simulink model "targetDice"  (R2020a)
settings: Solver=VariableStepAuto  StartTime=0.0  StopTime=20  RelTol=1e-3
model workspace (MAT data in the model file):
  d = [1  1  1  5  5  8; 2  2  3  3  6  6; 1  4  4  4  5  7; 2  2  6  6  7  8; 3  4  5  7  8  8]
  seed = 1234
libraries: simulink x1, rllib x1
settings Model: OrderedModelArguments=off  Creator=mtearle  LastModifiedBy=mtearle

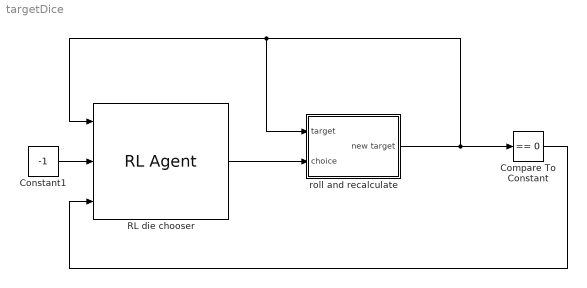
== system targetDice ==
  Compare To Constant : simulink/Logic and Bit Operations/Compare To Constant  relop===  const=0  OutDataTypeStr=boolean
  Constant1 : Constant  Value=-1
  RL die chooser : rllib/RL Agent  Agent=agent  ProvideReward=on  ProvideIsDone=on  ProvideCumRwd=off  TreatAsDirectFeedthrough=on  CollectLoggedSignals=on  CollectModelStates=on
  roll and recalculate : Subsystem
  wires:
  roll and recalculate/1(" new target") -> Compare To Constant/1, roll and recalculate/1(target), RL die chooser/1
  RL die chooser/1 -> roll and recalculate/2(choice)
  Constant1/1 -> RL die chooser/2
  Compare To Constant/1 -> RL die chooser/3

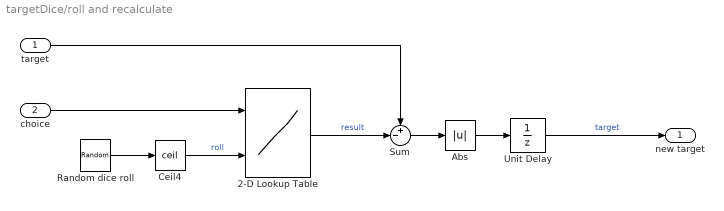
== system targetDice/roll and recalculate ==
  target : Inport
  choice : Inport  Port=2
  2-D Lookup Table : Lookup_n-D  BreakpointsSpecification=Even spacing  BreakpointsForDimension1=[1:3]  BreakpointsForDimension2=[1:3]  Table=d  InternalRulePriority=Speed  RndMeth=Simplest  InputSameDT=on
  Abs : Abs
  Ceil4 : Rounding  Operator=ceil
  Random dice roll : UniformRandomNumber  Minimum=0  Maximum=size(d,2)  Seed=seed  SampleTime=1
  Sum : Sum  Inputs=+-|
  Unit Delay : UnitDelay  InitialCondition=randi(20)  HasFrameUpgradeWarning=on
  " new target" : Outport
  wires:
  Sum/1 -> Abs/1
  Random dice roll/1 -> Ceil4/1
  Unit Delay/1 -> " new target"/1  "target"
  Ceil4/1 -> 2-D Lookup Table/2  "roll"
  2-D Lookup Table/1 -> Sum/2  "result"
  choice/1 -> 2-D Lookup Table/1
  Abs/1 -> Unit Delay/1
  target/1 -> Sum/1
